simulink model "Model2"  (R2018b)
settings: Solver=VariableStepAuto  StartTime=0.0  StopTime=10.0  RelTol=1e-3
values from neighbouring files (symbols this model uses):
  a = 0.9    [dane.m]
  b = 1.07    [dane.m]
  c = 0.2773    [dane.m]
  d = 0.0026    [dane.m]
  g = 9.81    [ABS.m]    (also in dane.m)
  Jw = 0.01    [ABS.m]    (also in dane.m)
  mv = 1200    [ABS.m]    (also in dane.m)
  rw = 0.28    [ABS.m]    (also in dane.m = 0.3)
settings Model: Creator=Kasia  LastModifiedBy=Kasia

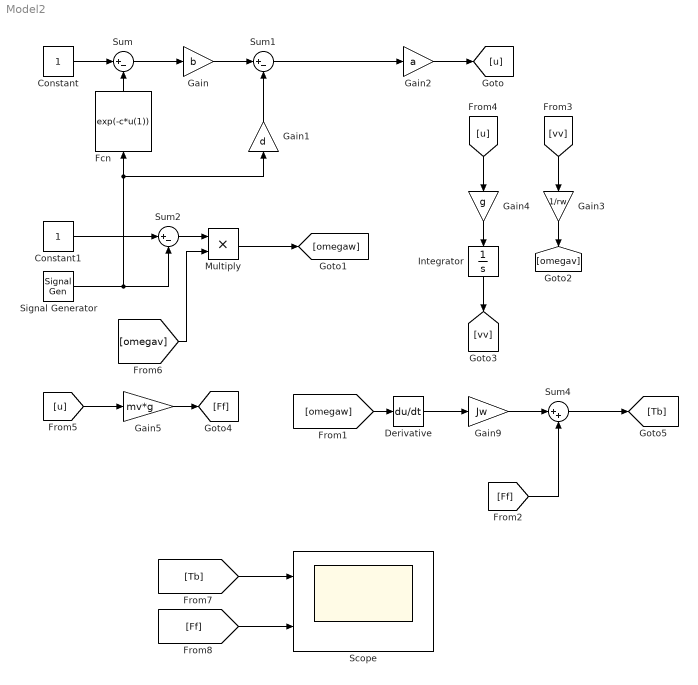
== system Model2 ==
  Constant : Constant
  Constant1 : Constant
  Derivative : Derivative
  Fcn : Fcn  Expr=exp(-c*u(1))
  Gain : Gain  Gain=b
  Gain1 : Gain  Gain=d
  Gain2 : Gain  Gain=a
  Gain3 : Gain  Gain=1/rw
  Gain4 : Gain  Gain=g
  Gain5 : Gain  Gain=mv*g
  Gain9 : Gain  Gain=Jw
  Integrator : Integrator
  Multiply : Product
  Scope : Scope  NumInputPorts=2
  Signal Generator : SignalGenerator  Units=rad/sec
  Sum : Sum  Inputs=|+-
  Sum1 : Sum  Inputs=|+-
  Sum2 : Sum  Inputs=|+-
  Sum4 : Sum  Inputs=|++
  wires:
  Signal Generator/1 -> Gain1/1, Fcn/1, Sum2/2
  Gain5/1 -> [Ff]
  Gain4/1 -> Integrator/1
  Gain1/1 -> Sum1/2
  Sum2/1 -> Multiply/1
  [vv] -> Gain3/1
  Integrator/1 -> [vv]
  Fcn/1 -> Sum/2
  Constant1/1 -> Sum2/1
  Gain3/1 -> [omegav]
  [u] -> Gain4/1
  [u] -> Gain5/1
  Multiply/1 -> [omegaw]
  Sum1/1 -> Gain2/1
  Gain2/1 -> [u]
  Gain/1 -> Sum1/1
  Sum/1 -> Gain/1
  Constant/1 -> Sum/1
  [omegaw] -> Derivative/1
  Derivative/1 -> Gain9/1
  Gain9/1 -> Sum4/1
  Sum4/1 -> [Tb]
  [Ff] -> Sum4/2
  [omegav] -> Multiply/2
  [Tb] -> Scope/1
  [Ff] -> Scope/2
